simulink model "SPGF_FSK_0000_R2019b"  (R2019b)
settings: Solver=ode3  SolverName=ode4  StartTime=0.0  StopTime=1.4  FixedStep=50e-6/50  RelTol=1e-3  EnableMultiTasking=on
undefined symbols (not defined in the file): D11, Delta
libraries: powerlib x2544, powerlib_meascontrol x204, simulink x24
(part 27 of 33)

== system SPGF_FSK_0000_R2019b/W52/concentrated ==
  Ccs/1 : powerlib/Elements/Series RLC Branch  LConnTagsString=__new0  RConnTagsString=__new0  BranchType=C  Resistance=190  Inductance=1e-3  SetiL0=off  InitialCurrent=0  Capacitance=-C_matrix(1,2)/2  Setx0=off  InitialVoltage=0  Measurements=None
  Ccs/2 : powerlib/Elements/Series RLC Branch  LConnTagsString=__new0  RConnTagsString=__new0  BranchType=C  Resistance=190  Inductance=1e-3  SetiL0=off  InitialCurrent=0  Capacitance=-C_matrix(1,2)/2  Setx0=off  InitialVoltage=0  Measurements=None
  Ccs2/1 : powerlib/Elements/Series RLC Branch  LConnTagsString=__new0  RConnTagsString=__new0  BranchType=C  Resistance=190  Inductance=1e-3  SetiL0=off  InitialCurrent=0  Capacitance=-C_matrix(3,4)/2  Setx0=off  InitialVoltage=0  Measurements=None
  Ccs2/2 : powerlib/Elements/Series RLC Branch  LConnTagsString=__new0  RConnTagsString=__new0  BranchType=C  Resistance=190  Inductance=1e-3  SetiL0=off  InitialCurrent=0  Capacitance=-C_matrix(3,4)/2  Setx0=off  InitialVoltage=0  Measurements=None
  Ccs2/3 : powerlib/Elements/Series RLC Branch  LConnTagsString=__new0  RConnTagsString=__new0  BranchType=R  Resistance=-Rg_matrix(3,4)*2  Inductance=1e-3  SetiL0=off  InitialCurrent=0  Capacitance=Rg_matrix(3,4)*2  Setx0=off  InitialVoltage=0  Measurements=None
  Ccs2/4 : powerlib/Elements/Series RLC Branch  LConnTagsString=__new0  RConnTagsString=__new0  BranchType=R  Resistance=-Rg_matrix(3,4)*2  Inductance=1e-3  SetiL0=off  InitialCurrent=0  Capacitance=Rg_matrix(3,4)*2  Setx0=off  InitialVoltage=0  Measurements=None
  Ccs3/1 : powerlib/Elements/Series RLC Branch  LConnTagsString=__new0  RConnTagsString=__new0  BranchType=C  Resistance=190  Inductance=1e-3  SetiL0=off  InitialCurrent=0  Capacitance=-C_matrix(5,6)/2  Setx0=off  InitialVoltage=0  Measurements=None
  Ccs3/2 : powerlib/Elements/Series RLC Branch  LConnTagsString=__new0  RConnTagsString=__new0  BranchType=C  Resistance=190  Inductance=1e-3  SetiL0=off  InitialCurrent=0  Capacitance=-C_matrix(5,6)/2  Setx0=off  InitialVoltage=0  Measurements=None
  Ccs3/3 : powerlib/Elements/Series RLC Branch  LConnTagsString=__new0  RConnTagsString=__new0  BranchType=R  Resistance=-Rg_matrix(5,6)*2  Inductance=1e-3  SetiL0=off  InitialCurrent=0  Capacitance=-C_matrix(5,6)/2  Setx0=off  InitialVoltage=0  Measurements=None
  Ccs3/4 : powerlib/Elements/Series RLC Branch  LConnTagsString=__new0  RConnTagsString=__new0  BranchType=R  Resistance=-Rg_matrix(5,6)*2  Inductance=1e-3  SetiL0=off  InitialCurrent=0  Capacitance=-C_matrix(5,6)/2  Setx0=off  InitialVoltage=0  Measurements=None
  Csg/2 : powerlib/Elements/Series RLC Branch  LConnTagsString=__new0  RConnTagsString=__new0  BranchType=C  Resistance=190  Inductance=1e-3  SetiL0=off  InitialCurrent=0  Capacitance=( C_matrix(1,2) + C_matrix(2,2) )/2  Setx0=off  InitialVoltage=0  Measurements=None
  Csg1/1 : powerlib/Elements/Series RLC Branch  LConnTagsString=__new0  RConnTagsString=__new0  BranchType=C  Resistance=190  Inductance=1e-3  SetiL0=off  InitialCurrent=0  Capacitance=( C_matrix(1,2) + C_matrix(2,2) )/2  Setx0=off  InitialVoltage=0  Measurements=None
  Csg2/1 : powerlib/Elements/Series RLC Branch  LConnTagsString=__new0  RConnTagsString=__new0  BranchType=C  Resistance=190  Inductance=1e-3  SetiL0=off  InitialCurrent=0  Capacitance=( C_matrix(3,4) + C_matrix(4,4) )/2  Setx0=off  InitialVoltage=0  Measurements=None
  Csg2/2 : powerlib/Elements/Series RLC Branch  LConnTagsString=__new0  RConnTagsString=__new0  BranchType=C  Resistance=190  Inductance=1e-3  SetiL0=off  InitialCurrent=0  Capacitance=( C_matrix(3,4) + C_matrix(4,4) )/2  Setx0=off  InitialVoltage=0  Measurements=None
  Csg3/1 : powerlib/Elements/Series RLC Branch  LConnTagsString=__new0  RConnTagsString=__new0  BranchType=C  Resistance=190  Inductance=1e-3  SetiL0=off  InitialCurrent=0  Capacitance=( C_matrix(5,6) + C_matrix(6,6) ) /2  Setx0=off  InitialVoltage=0  Measurements=None
  Csg3/2 : powerlib/Elements/Series RLC Branch  LConnTagsString=__new0  RConnTagsString=__new0  BranchType=C  Resistance=190  Inductance=1e-3  SetiL0=off  InitialCurrent=0  Capacitance=( C_matrix(5,6) + C_matrix(6,6) ) /2  Setx0=off  InitialVoltage=0  Measurements=None
  Ground{1..4} (4 alike) : powerlib/Elements/Ground  LConnTagsString=a
  RL : powerlib/Elements/Mutual Inductance  LConnTagsString=a|b|c|L4|L5|L6  RConnTagsString=A|B|C|R4|R5|R6  TypeOfMutual=Generalized mutual inductance  NumberOfWindings=6  SelfImpedance1=[1.1 1.1e-03]  SelfImpedance2=[ 1.1 1.1e-03]  ThreeWindings=on  SelfImpedance3=[ 1.1 1.1e-03]  MutualImpedance=[1.0 1.0e-03]  InductanceMatrix=L_matrix  ResistanceMatrix=R_matrix  Measurements=None
      settings: AttributesFormatString=\n
  Rcs*2 : powerlib/Elements/Series RLC Branch  LConnTagsString=__new0  RConnTagsString=__new0  BranchType=R  Resistance=-Rg_matrix(1,2)*2  Inductance=1e-3  SetiL0=off  InitialCurrent=0  Capacitance=Rg_matrix(1,2)*2  Setx0=off  InitialVoltage=0  Measurements=None
  Rgcs1/1 : powerlib/Elements/Series RLC Branch  LConnTagsString=__new0  RConnTagsString=__new0  BranchType=R  Resistance=-Rg_matrix(1,2)*2  Inductance=1e-3  SetiL0=off  InitialCurrent=0  Capacitance=Rg_matrix(1,2)*2  Setx0=off  InitialVoltage=0  Measurements=None
  Rgsg1/1 : powerlib/Elements/Series RLC Branch  LConnTagsString=__new0  RConnTagsString=__new0  BranchType=R  Resistance=(Rg_matrix(4,4)+Rg_matrix(3,4))*2  Inductance=1e-3  SetiL0=off  InitialCurrent=0  Capacitance=Rg_matrix(1,2)*2  Setx0=off  InitialVoltage=0  Measurements=None
  Rgsg1/2 : powerlib/Elements/Series RLC Branch  LConnTagsString=__new0  RConnTagsString=__new0  BranchType=R  Resistance=(Rg_matrix(2,2)+Rg_matrix(1,2))*2  Inductance=1e-3  SetiL0=off  InitialCurrent=0  Capacitance=Rg_matrix(1,2)*2  Setx0=off  InitialVoltage=0  Measurements=None
  Rgsg1/3 : powerlib/Elements/Series RLC Branch  LConnTagsString=__new0  RConnTagsString=__new0  BranchType=R  Resistance=(Rg_matrix(4,4)+Rg_matrix(3,4))*2  Inductance=1e-3  SetiL0=off  InitialCurrent=0  Capacitance=Rg_matrix(1,2)*2  Setx0=off  InitialVoltage=0  Measurements=None
  Rgsg1/4 : powerlib/Elements/Series RLC Branch  LConnTagsString=__new0  RConnTagsString=__new0  BranchType=R  Resistance=(Rg_matrix(2,2)+Rg_matrix(1,2))*2  Inductance=1e-3  SetiL0=off  InitialCurrent=0  Capacitance=Rg_matrix(1,2)*2  Setx0=off  InitialVoltage=0  Measurements=None
  Rsg*2 : powerlib/Elements/Series RLC Branch  LConnTagsString=__new0  RConnTagsString=__new0  BranchType=R  Resistance=(Rg_matrix(6,6)+Rg_matrix(5,6))*2  Inductance=1e-3  SetiL0=off  InitialCurrent=0  Capacitance=Rg_matrix(1,2)*2  Setx0=off  InitialVoltage=0  Measurements=None
  Rsg1/1 : powerlib/Elements/Series RLC Branch  LConnTagsString=__new0  RConnTagsString=__new0  BranchType=R  Resistance=(Rg_matrix(6,6)+Rg_matrix(5,6))*2  Inductance=1e-3  SetiL0=off  InitialCurrent=0  Capacitance=Rg_matrix(1,2)*2  Setx0=off  InitialVoltage=0  Measurements=None
  A : PMIOPort  Side=Left
  B : PMIOPort  Port=2  Side=Left
  C : PMIOPort  Port=3  Side=Left
  a : PMIOPort  Port=4  Side=Right
  b : PMIOPort  Port=5  Side=Right
  c : PMIOPort  Port=6  Side=Right
  connections:
  RL/LConn6 -- Ground3/LConn1 -- Rgsg1/2/LConn1 -- Csg/2/LConn1 -- Rcs*2/LConn1 -- Ccs/2/LConn1 -- RL/LConn2 -- RL/LConn4 -- Rgsg1/1/LConn1 -- Csg2/2/LConn1 -- Ccs2/3/LConn1 -- Ccs2/2/LConn1 -- Rsg*2/LConn1 -- Csg3/2/LConn1 -- Ccs3/3/LConn1 -- Ccs3/2/LConn1
  Rsg1/1/RConn1 -- Rgsg1/3/RConn1 -- Rgsg1/4/RConn1 -- Csg3/1/RConn1 -- Csg2/1/RConn1 -- Ground2/LConn1 -- Csg1/1/RConn1
  Rgsg1/3/LConn1 -- Ccs2/4/LConn1 -- Csg2/1/LConn1 -- Ccs2/1/LConn1 -- RL/RConn4 -- Rgsg1/4/LConn1 -- Rgcs1/1/LConn1 -- Csg1/1/LConn1 -- Ccs/1/LConn1 -- RL/RConn2 -- Ground4/LConn1 -- RL/RConn6 -- Ccs3/1/LConn1 -- Rsg1/1/LConn1 -- Ccs3/4/LConn1 -- Csg3/1/LConn1
  Rsg*2/RConn1 -- Rgsg1/1/RConn1 -- Rgsg1/2/RConn1 -- Csg3/2/RConn1 -- Csg2/2/RConn1 -- Ground1/LConn1 -- Csg/2/RConn1
  a/RConn1 -- RL/RConn1 -- Rgcs1/1/RConn1 -- Ccs/1/RConn1
  b/RConn1 -- RL/RConn3 -- Ccs2/4/RConn1 -- Ccs2/1/RConn1
  Ccs3/1/RConn1 -- c/RConn1 -- RL/RConn5 -- Ccs3/4/RConn1
  RL/LConn1 -- A/RConn1 -- Rcs*2/RConn1 -- Ccs/2/RConn1
  RL/LConn3 -- B/RConn1 -- Ccs2/3/RConn1 -- Ccs2/2/RConn1
  Ccs3/2/RConn1 -- C/RConn1 -- RL/LConn5 -- Ccs3/3/RConn1

== system SPGF_FSK_0000_R2019b/W53/DPL ==
  Ccs2/1 : powerlib/Elements/Series RLC Branch  LConnTagsString=__new0  RConnTagsString=__new0  BranchType=R  Resistance=-Rg_matrix(3,4)*2  Inductance=1e-3  SetiL0=off  InitialCurrent=0  Capacitance=Rg_matrix(3,4)*2  Setx0=off  InitialVoltage=0  Measurements=None
  Ccs2/3 : powerlib/Elements/Series RLC Branch  LConnTagsString=__new0  RConnTagsString=__new0  BranchType=R  Resistance=-Rg_matrix(3,4)*2  Inductance=1e-3  SetiL0=off  InitialCurrent=0  Capacitance=Rg_matrix(3,4)*2  Setx0=off  InitialVoltage=0  Measurements=None
  Ccs3/1 : powerlib/Elements/Series RLC Branch  LConnTagsString=__new0  RConnTagsString=__new0  BranchType=R  Resistance=-Rg_matrix(5,6)*2  Inductance=1e-3  SetiL0=off  InitialCurrent=0  Capacitance=-C_matrix(5,6)/2  Setx0=off  InitialVoltage=0  Measurements=None
  Ccs3/3 : powerlib/Elements/Series RLC Branch  LConnTagsString=__new0  RConnTagsString=__new0  BranchType=R  Resistance=-Rg_matrix(5,6)*2  Inductance=1e-3  SetiL0=off  InitialCurrent=0  Capacitance=-C_matrix(5,6)/2  Setx0=off  InitialVoltage=0  Measurements=None
  DPL : powerlib/Elements/Distributed Parameters Line  Phases=6  Length=LineLength  Frequency=Frequency  Resistance=R_matrix  Inductance=L_matrix  Capacitance=C_matrix  x1=[-7.5e-06 -1.54183560636282 0 0 0 0 0;-7e-06 -1.54227711389764 0 0 0 0 0;-6.5e-06 -1.5427185833783 0 0 0 0 0;-6e-06 -1.5431600147939 0 0 0 0 0;-5.5e-06 -1.54360140813356 0 0 0 0 0;-5e-06 -1.54404276338638 0 0 0 0 0;-4.5e-06 -1.54448408054147 0 0 0 0 0;-4e-06 -1.54492535958794 0 0 0 0 0;-3.5e-06 -1.54536660051491 0 0 0 0 0;-3e-06 -1.54580780331148 0 0 0 0 0;-2.5e-06 -1.54624896796678 0 0 0 0 0;-2e-06 -1.54669009446991 0 -12.1184330880716 0 0 0;-1.5e-06 -1.54713118281 5088.14933742732 -12.1219197812896 -2683.87508550843 4746.07026643471 0;-1e-06 -1.54757223297615 5089.56225063694 -12.1254061754113 -2684.62036287942 4745.64805376133 -8993.80208546917;-5e-07 -1.54801324495749 5090.97503826663 -12.1288922703505 -2685.36557401007 4745.22572399377 -8993.00169945208]  x2=[-7.5e-06 -1.54177439888293 0 0 0 0 0;-7e-06 -1.54221618808927 0 0 0 0 0;-6.5e-06 -1.54265793924295 0 0 0 0 0;-6e-06 -1.54309965233308 0 0 0 0 0;-5.5e-06 -1.54354132734875 0 0 0 0 0;-5e-06 -1.54398296427906 0 0 0 0 0;-4.5e-06 -1.54442456311312 0 0 0 0 0;-4e-06 -1.54486612384003 0 0 0 0 0;-3.5e-06 -1.5453076464489 0 0 0 0 0;-3e-06 -1.54574913092883 0 0 0 0 0;-2.5e-06 -1.54619057726893 0 0 0 0 0;-2e-06 -1.5466319854583 0 -12.1174441163831 0 0 0;-1.5e-06 -1.54707335548606 5088.61162249754 -12.1209335012858 -2684.11892964451 4747.16396717449 0;-1e-06 -1.54751468734132 5090.02486905971 -12.1244225871164 -2684.86438285087 4746.74173227726 -8995.87479039923;-5e-07 -1.54795598101318 5091.43799003055 -12.1279113737889 -2685.60976981087 4746.31938025886 -8995.07436221307]  x3=[-7.5e-06 -0.00538073782589089 0 0 0 0 0;-7e-06 -0.00538388219933964 0 0 0 0 0;-6.5e-06 -0.00538702643994642 0 0 0 0 0;-6e-06 -0.00539017054763365 0 0 0 0 0;-5.5e-06 -0.00539331452232375 0 0 0 0 0;-5e-06 -0.00539645836393916 0 0 0 0 0;-4.5e-06 -0.00539960207240229 0 0 0 0 0;-4e-06 -0.00540274564763558 0 0 0 0 0;-3.5e-06 -0.00540588908956146 0 0 0 0 0;-3e-06 -0.00540903239810238 0 0 0 0 0;-2.5e-06 -0.00541217557318077 0 0 0 0 0;-2e-06 -0.00541531861471909 0 -0.700013230034034 0 0 0;-1.5e-06 -0.00541846152263977 57.5957872318405 -0.700252773488419 -222.767391645066 432.465665177143 0;-1e-06 -0.00542160429686527 57.6182925325805 -0.700492299664759 -222.830475891123 432.428004367959 -162.228058382252;-5e-07 -0.00542474693731805 57.6407964116461 -0.700731808557144 -222.893554639059 432.390332889041 -162.217245837524]  x4=[-7.5e-06 -0.0147618097854623 0 0 0 0 0;-7e-06 -0.0147644504009928 0 0 0 0 0;-6.5e-06 -0.0147670906522252 0 0 0 0 0;-6e-06 -0.0147697305390942 0 0 0 0 0;-5.5e-06 -0.0147723700615347 0 0 0 0 0;-5e-06 -0.0147750092194815 0 0 0 0 0;-4.5e-06 -0.0147776480128697 0 0 0 0 0;-4e-06 -0.014780286441634 0 0 0 0 0;-3.5e-06 -0.0147829245057093 0 0 0 0 0;-3e-06 -0.0147855622050306 0 0 0 0 0;-2.5e-06 -0.0147881995395328 0 0 0 0 0;-2e-06 -0.0147908365091508 0 -0.756373897111339 0 0 0;-1.5e-06 -0.0147934731138195 70.4067235244733 -0.756553801145288 -218.988275314097 411.188287136 0;-1e-06 -0.0147961093534739 70.4197806186761 -0.756733686512019 -219.047922421474 411.150932538181 -101.711209086781;-5e-07 -0.0147987452280489 70.4328359753406 -0.756913553207096 -219.10756412406 411.113567795619 -101.698543550063]  x5=7.04416471370102e-06  V1=ones(3,3)  V2=ones(3,3)  I1=ones(3,3)  I2=ones(3,3)  nHarmo=1  Measurements=None  Decoupling=off  VsMag0=0  VrMag0=0  VsAngle0=0  VrAngle0=0  IsMag0=0  IrMag0=0  IsAngle0=0  IrAngle0=0
  Ground{1..4} (4 alike) : powerlib/Elements/Ground  LConnTagsString=a
  Rcs*1 : powerlib/Elements/Series RLC Branch  LConnTagsString=__new0  RConnTagsString=__new0  BranchType=R  Resistance=-Rg_matrix(1,2)*2  Inductance=1e-3  SetiL0=off  InitialCurrent=0  Capacitance=Rg_matrix(1,2)*2  Setx0=off  InitialVoltage=0  Measurements=None
  Rcs*2 : powerlib/Elements/Series RLC Branch  LConnTagsString=__new0  RConnTagsString=__new0  BranchType=R  Resistance=-Rg_matrix(1,2)*2  Inductance=1e-3  SetiL0=off  InitialCurrent=0  Capacitance=Rg_matrix(1,2)*2  Setx0=off  InitialVoltage=0  Measurements=None
  Rgsg1/1 : powerlib/Elements/Series RLC Branch  LConnTagsString=__new0  RConnTagsString=__new0  BranchType=R  Resistance=(Rg_matrix(4,4)+Rg_matrix(3,4))*2  Inductance=1e-3  SetiL0=off  InitialCurrent=0  Capacitance=Rg_matrix(1,2)*2  Setx0=off  InitialVoltage=0  Measurements=None
  Rgsg1/2 : powerlib/Elements/Series RLC Branch  LConnTagsString=__new0  RConnTagsString=__new0  BranchType=R  Resistance=(Rg_matrix(2,2)+Rg_matrix(1,2))*2  Inductance=1e-3  SetiL0=off  InitialCurrent=0  Capacitance=Rg_matrix(1,2)*2  Setx0=off  InitialVoltage=0  Measurements=None
  Rgsg1/3 : powerlib/Elements/Series RLC Branch  LConnTagsString=__new0  RConnTagsString=__new0  BranchType=R  Resistance=(Rg_matrix(4,4)+Rg_matrix(3,4))*2  Inductance=1e-3  SetiL0=off  InitialCurrent=0  Capacitance=Rg_matrix(1,2)*2  Setx0=off  InitialVoltage=0  Measurements=None
  Rgsg1/4 : powerlib/Elements/Series RLC Branch  LConnTagsString=__new0  RConnTagsString=__new0  BranchType=R  Resistance=(Rg_matrix(2,2)+Rg_matrix(1,2))*2  Inductance=1e-3  SetiL0=off  InitialCurrent=0  Capacitance=Rg_matrix(1,2)*2  Setx0=off  InitialVoltage=0  Measurements=None
  Rsg*1 : powerlib/Elements/Series RLC Branch  LConnTagsString=__new0  RConnTagsString=__new0  BranchType=R  Resistance=(Rg_matrix(6,6)+Rg_matrix(5,6))*2  Inductance=1e-3  SetiL0=off  InitialCurrent=0  Capacitance=Rg_matrix(1,2)*2  Setx0=off  InitialVoltage=0  Measurements=None
  Rsg*2 : powerlib/Elements/Series RLC Branch  LConnTagsString=__new0  RConnTagsString=__new0  BranchType=R  Resistance=(Rg_matrix(6,6)+Rg_matrix(5,6))*2  Inductance=1e-3  SetiL0=off  InitialCurrent=0  Capacitance=Rg_matrix(1,2)*2  Setx0=off  InitialVoltage=0  Measurements=None
  A : PMIOPort  Side=Left
  B : PMIOPort  Port=2  Side=Left
  C : PMIOPort  Port=3  Side=Left
  a : PMIOPort  Port=4  Side=Right
  b : PMIOPort  Port=5  Side=Right
  c : PMIOPort  Port=6  Side=Right
  connections:
  A/RConn1 -- DPL/LConn1 -- Rcs*2/RConn1
  B/RConn1 -- DPL/LConn3 -- Ccs2/3/RConn1
  C/RConn1 -- DPL/LConn5 -- Ccs3/3/RConn1
  Rgsg1/2/RConn1 -- Rsg*2/RConn1 -- Rgsg1/1/RConn1 -- Ground2/LConn1
  DPL/LConn2 -- Rcs*2/LConn1 -- Rgsg1/2/LConn1 -- DPL/LConn4 -- Ccs2/3/LConn1 -- Rgsg1/1/LConn1 -- DPL/LConn6 -- Rsg*2/LConn1 -- Ccs3/3/LConn1 -- Ground3/LConn1
  Rgsg1/3/RConn1 -- Rsg*1/RConn1 -- Rgsg1/4/RConn1 -- Ground1/LConn1
  Rgsg1/3/LConn1 -- Ccs2/1/LConn1 -- DPL/RConn4 -- DPL/RConn2 -- Rgsg1/4/LConn1 -- Rcs*1/LConn1 -- Rsg*1/LConn1 -- Ccs3/1/LConn1 -- DPL/RConn6 -- Ground4/LConn1
  Rcs*1/RConn1 -- DPL/RConn1 -- a/RConn1
  DPL/RConn3 -- Ccs2/1/RConn1 -- b/RConn1
  DPL/RConn5 -- Ccs3/1/RConn1 -- c/RConn1

== system SPGF_FSK_0000_R2019b/W53/Pi ==
  Ground{,1..8} (9 alike) : powerlib/Elements/Ground  LConnTagsString=a
  Series RLC Branch{,1..2,27..28,33} (6 alike) : powerlib/Elements/Series RLC Branch  LConnTagsString=__new0  RConnTagsString=__new0  BranchType=RL  Resistance=R/2  Inductance=L/2  SetiL0=off  InitialCurrent=0  Capacitance=1e-6  Setx0=off  InitialVoltage=0  Measurements=None
  Series RLC Branch{10..11,13,29..30,32} (6 alike) : powerlib/Elements/Series RLC Branch  LConnTagsString=__new0  RConnTagsString=__new0  BranchType=R  Resistance=Rfg*4  Inductance=L/2  SetiL0=off  InitialCurrent=0  Capacitance=1e-6  Setx0=off  InitialVoltage=0  Measurements=None
  Series RLC Branch{9,12,14,31,40..41} (6 alike) : powerlib/Elements/Series RLC Branch  LConnTagsString=__new0  RConnTagsString=__new0  BranchType=C  Resistance=R/2  Inductance=L/2  SetiL0=off  InitialCurrent=0  Capacitance=Cfg*0.25  Setx0=off  InitialVoltage=0  Measurements=None
  Series RLC Branch15 : powerlib/Elements/Series RLC Branch  LConnTagsString=__new0  RConnTagsString=__new0  BranchType=R  Resistance=Rfg*2  Inductance=L/2  SetiL0=off  InitialCurrent=0  Capacitance=1e-6  Setx0=off  InitialVoltage=0  Measurements=None
  Series RLC Branch16 : powerlib/Elements/Series RLC Branch  LConnTagsString=__new0  RConnTagsString=__new0  BranchType=R  Resistance=Rfg*2  Inductance=L/2  SetiL0=off  InitialCurrent=0  Capacitance=1e-6  Setx0=off  InitialVoltage=0  Measurements=None
  Series RLC Branch17 : powerlib/Elements/Series RLC Branch  LConnTagsString=__new0  RConnTagsString=__new0  BranchType=C  Resistance=R/2  Inductance=L/2  SetiL0=off  InitialCurrent=0  Capacitance=Cfg*0.5  Setx0=off  InitialVoltage=0  Measurements=None
  Series RLC Branch18 : powerlib/Elements/Series RLC Branch  LConnTagsString=__new0  RConnTagsString=__new0  BranchType=R  Resistance=Rfg*2  Inductance=L/2  SetiL0=off  InitialCurrent=0  Capacitance=1e-6  Setx0=off  InitialVoltage=0  Measurements=None
  Series RLC Branch19 : powerlib/Elements/Series RLC Branch  LConnTagsString=__new0  RConnTagsString=__new0  BranchType=C  Resistance=R/2  Inductance=L/2  SetiL0=off  InitialCurrent=0  Capacitance=Cfg*0.5  Setx0=off  InitialVoltage=0  Measurements=None
  Series RLC Branch20 : powerlib/Elements/Series RLC Branch  LConnTagsString=__new0  RConnTagsString=__new0  BranchType=C  Resistance=R/2  Inductance=L/2  SetiL0=off  InitialCurrent=0  Capacitance=Cmf*0.5  Setx0=off  InitialVoltage=0  Measurements=None
  Series RLC Branch21 : powerlib/Elements/Series RLC Branch  LConnTagsString=__new0  RConnTagsString=__new0  BranchType=R  Resistance=Rmf*2  Inductance=L/2  SetiL0=off  InitialCurrent=0  Capacitance=1e-6  Setx0=off  InitialVoltage=0  Measurements=None
  Series RLC Branch22 : powerlib/Elements/Series RLC Branch  LConnTagsString=__new0  RConnTagsString=__new0  BranchType=C  Resistance=R/2  Inductance=L/2  SetiL0=off  InitialCurrent=0  Capacitance=Cmf*0.5  Setx0=off  InitialVoltage=0  Measurements=None
  Series RLC Branch23 : powerlib/Elements/Series RLC Branch  LConnTagsString=__new0  RConnTagsString=__new0  BranchType=R  Resistance=Rmf*2  Inductance=L/2  SetiL0=off  InitialCurrent=0  Capacitance=1e-6  Setx0=off  InitialVoltage=0  Measurements=None
  Series RLC Branch24 : powerlib/Elements/Series RLC Branch  LConnTagsString=__new0  RConnTagsString=__new0  BranchType=C  Resistance=R/2  Inductance=L/2  SetiL0=off  InitialCurrent=0  Capacitance=Cmf*0.5  Setx0=off  InitialVoltage=0  Measurements=None
  Series RLC Branch25 : powerlib/Elements/Series RLC Branch  LConnTagsString=__new0  RConnTagsString=__new0  BranchType=R  Resistance=Rmf*2  Inductance=L/2  SetiL0=off  InitialCurrent=0  Capacitance=1e-6  Setx0=off  InitialVoltage=0  Measurements=None
  Series RLC Branch26 : powerlib/Elements/Series RLC Branch  LConnTagsString=__new0  RConnTagsString=__new0  BranchType=C  Resistance=R/2  Inductance=L/2  SetiL0=off  InitialCurrent=0  Capacitance=Cfg*0.5  Setx0=off  InitialVoltage=0  Measurements=None
  Series RLC Branch{3,5,7,34,36,38} (6 alike) : powerlib/Elements/Series RLC Branch  LConnTagsString=__new0  RConnTagsString=__new0  BranchType=C  Resistance=R/2  Inductance=L/2  SetiL0=off  InitialCurrent=0  Capacitance=Cmf*0.25  Setx0=off  InitialVoltage=0  Measurements=None
  Series RLC Branch{4,6,8,35,37,39} (6 alike) : powerlib/Elements/Series RLC Branch  LConnTagsString=__new0  RConnTagsString=__new0  BranchType=R  Resistance=Rmf*4  Inductance=L/2  SetiL0=off  InitialCurrent=0  Capacitance=1e-6  Setx0=off  InitialVoltage=0  Measurements=None
  A : PMIOPort  Side=Left
  B : PMIOPort  Port=2  Side=Left
  C : PMIOPort  Port=3  Side=Left
  a : PMIOPort  Port=4  Side=Right
  b : PMIOPort  Port=5  Side=Right
  c : PMIOPort  Port=6  Side=Right
  connections:
  Series RLC Branch12/LConn1 -- Series RLC Branch11/LConn1 -- Series RLC Branch5/LConn1 -- Series RLC Branch6/LConn1 -- B/RConn1 -- Series RLC Branch4/RConn1 -- Series RLC Branch3/RConn1 -- Series RLC Branch1/LConn1
  Series RLC Branch13/LConn1 -- A/RConn1 -- Series RLC Branch4/LConn1 -- Series RLC Branch3/LConn1 -- Series RLC Branch7/LConn1 -- Series RLC Branch8/LConn1 -- Series RLC Branch/LConn1 -- Series RLC Branch14/LConn1
  Series RLC Branch9/LConn1 -- Series RLC Branch2/LConn1 -- Series RLC Branch8/RConn1 -- Series RLC Branch7/RConn1 -- C/RConn1 -- Series RLC Branch5/RConn1 -- Series RLC Branch6/RConn1 -- Series RLC Branch10/LConn1
  Series RLC Branch9/RConn1 -- Ground/LConn1 -- Series RLC Branch10/RConn1
  Series RLC Branch12/RConn1 -- Series RLC Branch11/RConn1 -- Ground1/LConn1
  Series RLC Branch13/RConn1 -- Series RLC Branch14/RConn1 -- Ground2/LConn1
  Series RLC Branch17/LConn1 -- Series RLC Branch16/LConn1 -- Series RLC Branch28/LConn1 -- Series RLC Branch1/RConn1 -- Series RLC Branch23/LConn1 -- Series RLC Branch22/LConn1 -- Series RLC Branch20/RConn1 -- Series RLC Branch21/RConn1
  Series RLC Branch21/LConn1 -- Series RLC Branch20/LConn1 -- Series RLC Branch/RConn1 -- Series RLC Branch27/LConn1 -- Series RLC Branch19/LConn1 -- Series RLC Branch18/LConn1 -- Series RLC Branch24/LConn1 -- Series RLC Branch25/LConn1
  Series RLC Branch26/LConn1 -- Series RLC Branch15/LConn1 -- Series RLC Branch2/RConn1 -- Series RLC Branch33/LConn1 -- Series RLC Branch25/RConn1 -- Series RLC Branch24/RConn1 -- Series RLC Branch22/RConn1 -- Series RLC Branch23/RConn1
  Series RLC Branch26/RConn1 -- Series RLC Branch15/RConn1 -- Ground3/LConn1
  Ground4/LConn1 -- Series RLC Branch17/RConn1 -- Series RLC Branch16/RConn1
  Ground5/LConn1 -- Series RLC Branch18/RConn1 -- Series RLC Branch19/RConn1
  Series RLC Branch31/LConn1 -- b/RConn1 -- Series RLC Branch35/RConn1 -- Series RLC Branch34/RConn1 -- Series RLC Branch36/LConn1 -- Series RLC Branch37/LConn1 -- Series RLC Branch28/RConn1 -- Series RLC Branch30/LConn1
  Series RLC Branch34/LConn1 -- a/RConn1 -- Series RLC Branch41/LConn1 -- Series RLC Branch32/LConn1 -- Series RLC Branch38/LConn1 -- Series RLC Branch39/LConn1 -- Series RLC Branch27/RConn1 -- Series RLC Branch35/LConn1
  Series RLC Branch29/LConn1 -- Series RLC Branch36/RConn1 -- Series RLC Branch37/RConn1 -- c/RConn1 -- Series RLC Branch39/RConn1 -- Series RLC Branch38/RConn1 -- Series RLC Branch33/RConn1 -- Series RLC Branch40/LConn1
  Series RLC Branch29/RConn1 -- Series RLC Branch40/RConn1 -- Ground6/LConn1
  Series RLC Branch31/RConn1 -- Series RLC Branch30/RConn1 -- Ground7/LConn1
  Series RLC Branch32/RConn1 -- Series RLC Branch41/RConn1 -- Ground8/LConn1

== system SPGF_FSK_0000_R2019b/W53/Q ==
  breaker : Subsystem  Commented=on  mask{SwitchA=off, SwitchB=off, SwitchC=off, InitialStatus=[1 1 1], BreakerResistance=0.0001, SnubberResistance=1e6, SnubberCapacitance=inf, TransitionTimes=[0.5 0.7], ShiftTimes=[0 0 0]}
      mask prompts: SwitchA "Switching of phase A"; SwitchB "Switching of phase B"; SwitchC "Switching of phase C"; InitialStatus "Initial status of phase breaker [A, B, C]"; BreakerResistance "Breaker resistance Ron (ohms) :"; SnubberResistance "Snubbers resistance Rp (ohms) :"; SnubberCapacitance "Snubbers capacitance Cp (F) :"; TransitionTimes "Transition times (s) :"; ShiftTimes "Time differences for switch [tA, tB, tC] (s) :"
      mask init: same as SPGF_FSK_0000_R2019b/Feed/Q/breaker
      mask Display:
      | % port_label('input',1,'Iabc');
      | 
      | port_label('lconn',1,'A');
      | port_label('lconn',2,'B');
      | port_label('lconn',3,'C');
      | 
      | port_label('rconn',1,'a');
      | port_label('rconn',2,'b');
      | port_label('rconn',3,'c');
      | 
      | disp('   Q    ');
  meas : Subsystem
  shunt : Subsystem
  A : PMIOPort  Side=Right
  B : PMIOPort  Port=2  Side=Right
  C : PMIOPort  Port=3  Side=Right
  a : PMIOPort  Port=4  Side=Left
  b : PMIOPort  Port=5  Side=Left
  c : PMIOPort  Port=6  Side=Left
  connections:
  shunt/LConn3 -- C/RConn1 -- breaker/LConn3
  shunt/LConn2 -- B/RConn1 -- breaker/LConn2
  A/RConn1 -- shunt/LConn1 -- breaker/LConn1
  meas/RConn1 -- a/RConn1
  meas/RConn2 -- b/RConn1
  meas/RConn3 -- c/RConn1
  meas/LConn3 -- breaker/RConn3 -- shunt/RConn3
  meas/LConn2 -- breaker/RConn2 -- shunt/RConn2
  meas/LConn1 -- breaker/RConn1 -- shunt/RConn1

== system SPGF_FSK_0000_R2019b/W53/concentrated ==
  Ccs/1 : powerlib/Elements/Series RLC Branch  LConnTagsString=__new0  RConnTagsString=__new0  BranchType=C  Resistance=190  Inductance=1e-3  SetiL0=off  InitialCurrent=0  Capacitance=-C_matrix(1,2)/2  Setx0=off  InitialVoltage=0  Measurements=None
  Ccs/2 : powerlib/Elements/Series RLC Branch  LConnTagsString=__new0  RConnTagsString=__new0  BranchType=C  Resistance=190  Inductance=1e-3  SetiL0=off  InitialCurrent=0  Capacitance=-C_matrix(1,2)/2  Setx0=off  InitialVoltage=0  Measurements=None
  Ccs2/1 : powerlib/Elements/Series RLC Branch  LConnTagsString=__new0  RConnTagsString=__new0  BranchType=C  Resistance=190  Inductance=1e-3  SetiL0=off  InitialCurrent=0  Capacitance=-C_matrix(3,4)/2  Setx0=off  InitialVoltage=0  Measurements=None
  Ccs2/2 : powerlib/Elements/Series RLC Branch  LConnTagsString=__new0  RConnTagsString=__new0  BranchType=C  Resistance=190  Inductance=1e-3  SetiL0=off  InitialCurrent=0  Capacitance=-C_matrix(3,4)/2  Setx0=off  InitialVoltage=0  Measurements=None
  Ccs2/3 : powerlib/Elements/Series RLC Branch  LConnTagsString=__new0  RConnTagsString=__new0  BranchType=R  Resistance=-Rg_matrix(3,4)*2  Inductance=1e-3  SetiL0=off  InitialCurrent=0  Capacitance=Rg_matrix(3,4)*2  Setx0=off  InitialVoltage=0  Measurements=None
  Ccs2/4 : powerlib/Elements/Series RLC Branch  LConnTagsString=__new0  RConnTagsString=__new0  BranchType=R  Resistance=-Rg_matrix(3,4)*2  Inductance=1e-3  SetiL0=off  InitialCurrent=0  Capacitance=Rg_matrix(3,4)*2  Setx0=off  InitialVoltage=0  Measurements=None
  Ccs3/1 : powerlib/Elements/Series RLC Branch  LConnTagsString=__new0  RConnTagsString=__new0  BranchType=C  Resistance=190  Inductance=1e-3  SetiL0=off  InitialCurrent=0  Capacitance=-C_matrix(5,6)/2  Setx0=off  InitialVoltage=0  Measurements=None
  Ccs3/2 : powerlib/Elements/Series RLC Branch  LConnTagsString=__new0  RConnTagsString=__new0  BranchType=C  Resistance=190  Inductance=1e-3  SetiL0=off  InitialCurrent=0  Capacitance=-C_matrix(5,6)/2  Setx0=off  InitialVoltage=0  Measurements=None
  Ccs3/3 : powerlib/Elements/Series RLC Branch  LConnTagsString=__new0  RConnTagsString=__new0  BranchType=R  Resistance=-Rg_matrix(5,6)*2  Inductance=1e-3  SetiL0=off  InitialCurrent=0  Capacitance=-C_matrix(5,6)/2  Setx0=off  InitialVoltage=0  Measurements=None
  Ccs3/4 : powerlib/Elements/Series RLC Branch  LConnTagsString=__new0  RConnTagsString=__new0  BranchType=R  Resistance=-Rg_matrix(5,6)*2  Inductance=1e-3  SetiL0=off  InitialCurrent=0  Capacitance=-C_matrix(5,6)/2  Setx0=off  InitialVoltage=0  Measurements=None
  Csg/2 : powerlib/Elements/Series RLC Branch  LConnTagsString=__new0  RConnTagsString=__new0  BranchType=C  Resistance=190  Inductance=1e-3  SetiL0=off  InitialCurrent=0  Capacitance=( C_matrix(1,2) + C_matrix(2,2) )/2  Setx0=off  InitialVoltage=0  Measurements=None
  Csg1/1 : powerlib/Elements/Series RLC Branch  LConnTagsString=__new0  RConnTagsString=__new0  BranchType=C  Resistance=190  Inductance=1e-3  SetiL0=off  InitialCurrent=0  Capacitance=( C_matrix(1,2) + C_matrix(2,2) )/2  Setx0=off  InitialVoltage=0  Measurements=None
  Csg2/1 : powerlib/Elements/Series RLC Branch  LConnTagsString=__new0  RConnTagsString=__new0  BranchType=C  Resistance=190  Inductance=1e-3  SetiL0=off  InitialCurrent=0  Capacitance=( C_matrix(3,4) + C_matrix(4,4) )/2  Setx0=off  InitialVoltage=0  Measurements=None
  Csg2/2 : powerlib/Elements/Series RLC Branch  LConnTagsString=__new0  RConnTagsString=__new0  BranchType=C  Resistance=190  Inductance=1e-3  SetiL0=off  InitialCurrent=0  Capacitance=( C_matrix(3,4) + C_matrix(4,4) )/2  Setx0=off  InitialVoltage=0  Measurements=None
  Csg3/1 : powerlib/Elements/Series RLC Branch  LConnTagsString=__new0  RConnTagsString=__new0  BranchType=C  Resistance=190  Inductance=1e-3  SetiL0=off  InitialCurrent=0  Capacitance=( C_matrix(5,6) + C_matrix(6,6) ) /2  Setx0=off  InitialVoltage=0  Measurements=None
  Csg3/2 : powerlib/Elements/Series RLC Branch  LConnTagsString=__new0  RConnTagsString=__new0  BranchType=C  Resistance=190  Inductance=1e-3  SetiL0=off  InitialCurrent=0  Capacitance=( C_matrix(5,6) + C_matrix(6,6) ) /2  Setx0=off  InitialVoltage=0  Measurements=None
  Ground{1..4} (4 alike) : powerlib/Elements/Ground  LConnTagsString=a
  RL : powerlib/Elements/Mutual Inductance  LConnTagsString=a|b|c|L4|L5|L6  RConnTagsString=A|B|C|R4|R5|R6  TypeOfMutual=Generalized mutual inductance  NumberOfWindings=6  SelfImpedance1=[1.1 1.1e-03]  SelfImpedance2=[ 1.1 1.1e-03]  ThreeWindings=on  SelfImpedance3=[ 1.1 1.1e-03]  MutualImpedance=[1.0 1.0e-03]  InductanceMatrix=L_matrix  ResistanceMatrix=R_matrix  Measurements=None
      settings: AttributesFormatString=\n
  Rcs*2 : powerlib/Elements/Series RLC Branch  LConnTagsString=__new0  RConnTagsString=__new0  BranchType=R  Resistance=-Rg_matrix(1,2)*2  Inductance=1e-3  SetiL0=off  InitialCurrent=0  Capacitance=Rg_matrix(1,2)*2  Setx0=off  InitialVoltage=0  Measurements=None
  Rgcs1/1 : powerlib/Elements/Series RLC Branch  LConnTagsString=__new0  RConnTagsString=__new0  BranchType=R  Resistance=-Rg_matrix(1,2)*2  Inductance=1e-3  SetiL0=off  InitialCurrent=0  Capacitance=Rg_matrix(1,2)*2  Setx0=off  InitialVoltage=0  Measurements=None
  Rgsg1/1 : powerlib/Elements/Series RLC Branch  LConnTagsString=__new0  RConnTagsString=__new0  BranchType=R  Resistance=(Rg_matrix(4,4)+Rg_matrix(3,4))*2  Inductance=1e-3  SetiL0=off  InitialCurrent=0  Capacitance=Rg_matrix(1,2)*2  Setx0=off  InitialVoltage=0  Measurements=None
  Rgsg1/2 : powerlib/Elements/Series RLC Branch  LConnTagsString=__new0  RConnTagsString=__new0  BranchType=R  Resistance=(Rg_matrix(2,2)+Rg_matrix(1,2))*2  Inductance=1e-3  SetiL0=off  InitialCurrent=0  Capacitance=Rg_matrix(1,2)*2  Setx0=off  InitialVoltage=0  Measurements=None
  Rgsg1/3 : powerlib/Elements/Series RLC Branch  LConnTagsString=__new0  RConnTagsString=__new0  BranchType=R  Resistance=(Rg_matrix(4,4)+Rg_matrix(3,4))*2  Inductance=1e-3  SetiL0=off  InitialCurrent=0  Capacitance=Rg_matrix(1,2)*2  Setx0=off  InitialVoltage=0  Measurements=None
  Rgsg1/4 : powerlib/Elements/Series RLC Branch  LConnTagsString=__new0  RConnTagsString=__new0  BranchType=R  Resistance=(Rg_matrix(2,2)+Rg_matrix(1,2))*2  Inductance=1e-3  SetiL0=off  InitialCurrent=0  Capacitance=Rg_matrix(1,2)*2  Setx0=off  InitialVoltage=0  Measurements=None
  Rsg*2 : powerlib/Elements/Series RLC Branch  LConnTagsString=__new0  RConnTagsString=__new0  BranchType=R  Resistance=(Rg_matrix(6,6)+Rg_matrix(5,6))*2  Inductance=1e-3  SetiL0=off  InitialCurrent=0  Capacitance=Rg_matrix(1,2)*2  Setx0=off  InitialVoltage=0  Measurements=None
  Rsg1/1 : powerlib/Elements/Series RLC Branch  LConnTagsString=__new0  RConnTagsString=__new0  BranchType=R  Resistance=(Rg_matrix(6,6)+Rg_matrix(5,6))*2  Inductance=1e-3  SetiL0=off  InitialCurrent=0  Capacitance=Rg_matrix(1,2)*2  Setx0=off  InitialVoltage=0  Measurements=None
  A : PMIOPort  Side=Left
  B : PMIOPort  Port=2  Side=Left
  C : PMIOPort  Port=3  Side=Left
  a : PMIOPort  Port=4  Side=Right
  b : PMIOPort  Port=5  Side=Right
  c : PMIOPort  Port=6  Side=Right
  connections:
  RL/LConn6 -- Ground3/LConn1 -- Rgsg1/2/LConn1 -- Csg/2/LConn1 -- Rcs*2/LConn1 -- Ccs/2/LConn1 -- RL/LConn2 -- RL/LConn4 -- Rgsg1/1/LConn1 -- Csg2/2/LConn1 -- Ccs2/3/LConn1 -- Ccs2/2/LConn1 -- Rsg*2/LConn1 -- Csg3/2/LConn1 -- Ccs3/3/LConn1 -- Ccs3/2/LConn1
  Rsg1/1/RConn1 -- Rgsg1/3/RConn1 -- Rgsg1/4/RConn1 -- Csg3/1/RConn1 -- Csg2/1/RConn1 -- Ground2/LConn1 -- Csg1/1/RConn1
  Rgsg1/3/LConn1 -- Ccs2/4/LConn1 -- Csg2/1/LConn1 -- Ccs2/1/LConn1 -- RL/RConn4 -- Rgsg1/4/LConn1 -- Rgcs1/1/LConn1 -- Csg1/1/LConn1 -- Ccs/1/LConn1 -- RL/RConn2 -- Ground4/LConn1 -- RL/RConn6 -- Ccs3/1/LConn1 -- Rsg1/1/LConn1 -- Ccs3/4/LConn1 -- Csg3/1/LConn1
  Rsg*2/RConn1 -- Rgsg1/1/RConn1 -- Rgsg1/2/RConn1 -- Csg3/2/RConn1 -- Csg2/2/RConn1 -- Ground1/LConn1 -- Csg/2/RConn1
  a/RConn1 -- RL/RConn1 -- Rgcs1/1/RConn1 -- Ccs/1/RConn1
  b/RConn1 -- RL/RConn3 -- Ccs2/4/RConn1 -- Ccs2/1/RConn1
  Ccs3/1/RConn1 -- c/RConn1 -- RL/RConn5 -- Ccs3/4/RConn1
  RL/LConn1 -- A/RConn1 -- Rcs*2/RConn1 -- Ccs/2/RConn1
  RL/LConn3 -- B/RConn1 -- Ccs2/3/RConn1 -- Ccs2/2/RConn1
  Ccs3/2/RConn1 -- C/RConn1 -- RL/LConn5 -- Ccs3/3/RConn1
